simulink library "changeDetector"  (R2018b)
settings: Solver=VariableStepAuto  StartTime=0.0  StopTime=10.0  RelTol=1e-3
settings Model: Creator=muralikarnam  LastModifiedBy=muralikarnam

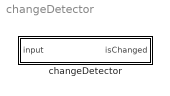
== system changeDetector ==
  changeDetector : Subsystem

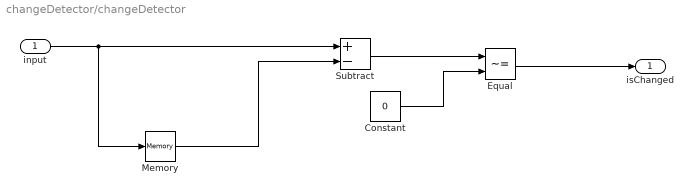
== system changeDetector/changeDetector ==
  input : Inport  PortDimensions=1
  Constant : Constant  Value=0
  Equal : RelationalOperator  Operator=~=  OutDataTypeStr=boolean  RndMeth=Simplest
  Memory : Memory
  Subtract : Sum  Inputs=+-
  "isChanged " : Outport  OutDataTypeStr=boolean  PortDimensions=1
  wires:
  input/1 -> Memory/1, Subtract/1
  Memory/1 -> Subtract/2
  Subtract/1 -> Equal/1
  Constant/1 -> Equal/2
  Equal/1 -> "isChanged "/1
